simulink model "C01A_DC_MotorEquation"  (R2024b)
settings: Solver=VariableStepAuto  StartTime=0.0  StopTime=0.2  RelTol=1e-3
undefined symbols (not defined in the file or in its folder): b, Cn, J, Km, L, R, RadToRpm, Tsample
settings Model: Creator=Davide  LastModifiedBy=Utente
settings DataIOCC: ReturnWorkspaceOutputs=off
settings OptimizationCC: ReuseModelBlockBuffer=off
settings RTWCC: GPUComputeCapability=3.5

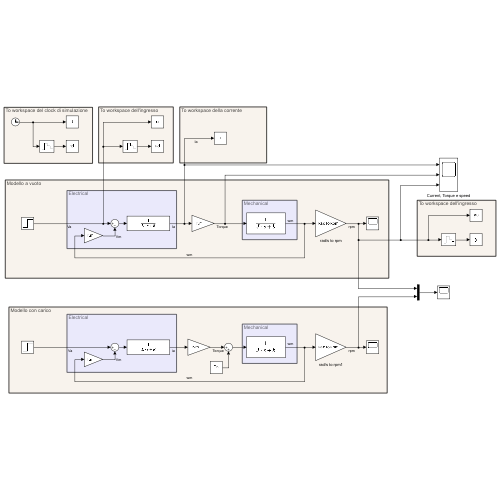
[thumbnail: Simulink's stored preview of the top-level diagram]
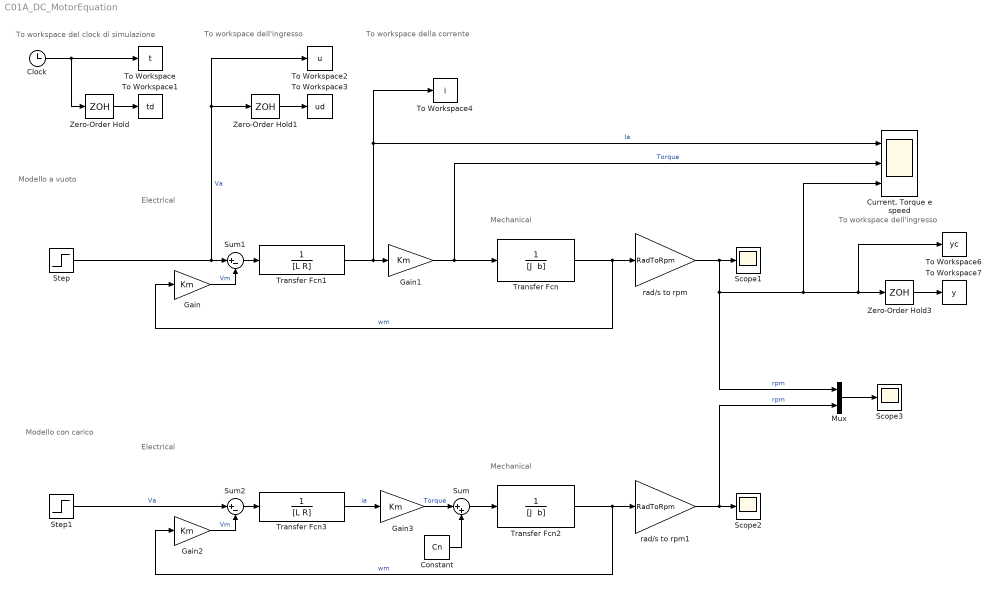
== system C01A_DC_MotorEquation ==
  note: To workspace dell'ingresso
  note: To workspace del clock di simulazione
  note: Modello a vuoto
  note: Modello con carico
  note: Electrical
  note: Mechanical
  note: Mechanical
  note: Electrical
  note: To workspace della corrente
  note: To workspace dell'ingresso
  Clock : Clock
  Constant : Constant  Value=Cn
  "Current, Torque e speed" : Scope  NumInputPorts=3
  Gain{,1..3} (4 alike) : Gain  Gain=Km
  Mux : Mux  Inputs=2
  Scope1 : Scope
  Scope2 : Scope
  Scope3 : Scope
  Step : Step  Time=0  After=24  SampleTime=0
  Step1 : Step  Time=0  After=24  SampleTime=0
  Sum : Sum  Inputs=|++
  Sum1 : Sum  Inputs=|+-
  Sum2 : Sum  Inputs=|+-
  To Workspace : ToWorkspace  VariableName=t  SampleTime=-1
  To Workspace1 : ToWorkspace  VariableName=td  SampleTime=-1
  To Workspace2 : ToWorkspace  VariableName=u  SampleTime=-1
  To Workspace3 : ToWorkspace  VariableName=ud  SampleTime=-1
  To Workspace4 : ToWorkspace  VariableName=i  SampleTime=-1
  To Workspace6 : ToWorkspace  VariableName=yc  SampleTime=-1
  To Workspace7 : ToWorkspace  VariableName=y  SampleTime=-1
  Transfer Fcn : TransferFcn  Denominator="[J  b]"
  Transfer Fcn1 : TransferFcn  Denominator=[L R]
  Transfer Fcn2 : TransferFcn  Denominator="[J  b]"
  Transfer Fcn3 : TransferFcn  Denominator=[L R]
  Zero-Order Hold : ZeroOrderHold  SampleTime=Tsample
  Zero-Order Hold1 : ZeroOrderHold  SampleTime=Tsample
  Zero-Order Hold3 : ZeroOrderHold  SampleTime=Tsample
  rad/s to rpm : Gain  Gain=RadToRpm  SaturateOnIntegerOverflow=on  OutDataTypeStr=Inherit: Same as input  ParamDataTypeStr=Inherit: Same as input
  rad/s to rpm1 : Gain  Gain=RadToRpm  SaturateOnIntegerOverflow=on  OutDataTypeStr=Inherit: Same as input  ParamDataTypeStr=Inherit: Same as input
  wires:
  rad/s to rpm/1 -> Mux/1, "Current, Torque e speed"/3, To Workspace6/1, Zero-Order Hold3/1, Scope1/1  "rpm"
  Transfer Fcn/1 -> rad/s to rpm/1, Gain/1  "wm"
  Sum1/1 -> Transfer Fcn1/1
  Gain/1 -> Sum1/2  "Vm"
  Step/1 -> Zero-Order Hold1/1, To Workspace2/1, Sum1/1  "Va"
  Gain1/1 -> "Current, Torque e speed"/2, Transfer Fcn/1  "Torque"
  rad/s to rpm1/1 -> Mux/2, Scope2/1  "rpm"
  Sum2/1 -> Transfer Fcn3/1
  Gain2/1 -> Sum2/2  "Vm"
  Transfer Fcn2/1 -> rad/s to rpm1/1, Gain2/1  "wm"
  Transfer Fcn3/1 -> Gain3/1  "ia"
  Step1/1 -> Sum2/1  "Va"
  Gain3/1 -> Sum/1  "Torque"
  Constant/1 -> Sum/2
  Mux/1 -> Scope3/1
  Sum/1 -> Transfer Fcn2/1
  Clock/1 -> Zero-Order Hold/1, To Workspace/1
  Zero-Order Hold/1 -> To Workspace1/1
  Zero-Order Hold1/1 -> To Workspace3/1
  Transfer Fcn1/1 -> "Current, Torque e speed"/1, To Workspace4/1, Gain1/1  "Ia"
  Zero-Order Hold3/1 -> To Workspace7/1
